simulink model "LAB2_BRUSHED_DC_MOTOR"  (R2023a)
settings: Solver=FixedStepAuto  StartTime=0.0  StopTime=inf  FixedStep=1/200  RelTol=1e-3  EnableMultiTasking=on
undefined symbols (not defined in the file): Dir, ena, freq, LF, pwm
libraries: instrumentseriallib x4, simulink x2, hdlsllib x1
settings Model: PacingRate=10  Creator=User  LastModifiedBy=User
settings SolverCC: AllowMultiTaskInputOutput=on  ConcurrentTasks=on  AutoInsertRateTranBlk=on

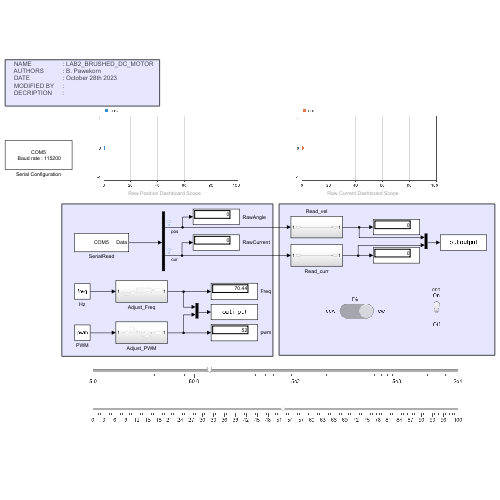
[thumbnail: Simulink's stored preview of the top-level diagram]
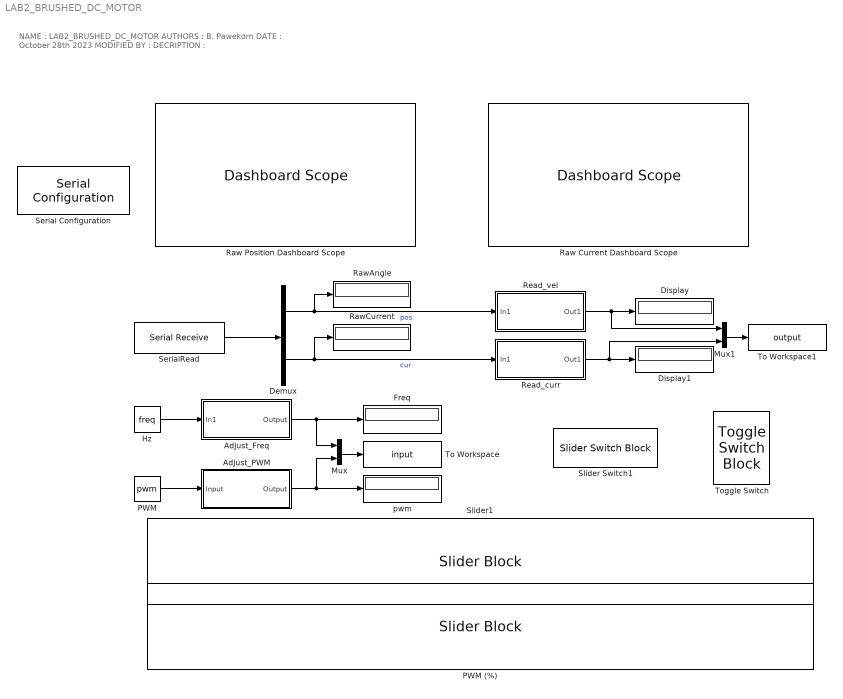
== system LAB2_BRUSHED_DC_MOTOR ==
  note: NAME                  : LAB2_BRUSHED_DC_MOTOR
      |     AUTHORS           : B. Pawekorn
      |     DATE                   : October 28th 2023
      |     MODIFIED BY     :
      |     DECRIPTION      :
  Adjust_Freq : Subsystem
  Adjust_PWM : Subsystem
  Demux : Demux  Outputs=2
  Display : Display
  Display1 : Display
  Freq : Display
  Hz : Constant  Value=freq  OutDataTypeStr=double
  Mux : Mux  Inputs=2
  Mux1 : Mux  Inputs=2
  PWM : Constant  Value=pwm  OutDataTypeStr=uint8
  PWM (%) : SliderBlock  LabelPosition=Hide
  Raw Current Dashboard Scope : DashboardScope  Ymin=0  Ymax=300  UpdateMode=Scroll
  Raw Position Dashboard Scope : DashboardScope  Ymin=0  Ymax=300  UpdateMode=Scroll
  RawAngle : Display
  RawCurrent : Display
  Read_curr : Subsystem
  Read_vel : Subsystem
  Serial Configuration : instrumentseriallib/Serial Configuration  Priority=-200000  PortSel=COM5  Port=COM5  ComPort=COM5  BaudRate=115200  DataBits=8  Parity=none  StopBits=1  ByteOrder=little-endian  FlowControl=none  Timeout=10  SimulateUsing=Interpreted execution  BlockInModel=on  aMode=1
      settings: LibrarySourceBlock=c2000lib/Host Communication/Serial Configuration
  SerialRead : instrumentseriallib/Serial Receive  Priority=1  PortSel=COM5  Port=COM5  ComPort=COM5  DataType=uint16  SaveDataType=uint8  ToggleHeader=on  Header=[69]  ToggleTerminator=on  Terminator=LF ('\n')  CustomTerminator=[]  InputFormat=Column major  ToggleDataSize=on  DataSize=[2]  EnableBlockingMode=on  ActionDataUnavailable=Output last received value  ActionWhenDataUnavailable=Output last received value  CustomValue=0  SampleTime=-1  SimulateUsing=Interpreted execution  BlockInModel=on  aMode=1
  Slider Switch1 : SliderSwitchBlock
      settings: Values={{'ccw', 'cw'}, [1 2]}
  Slider1 : SliderBlock  LabelPosition=Hide  ScaleMin=5  ScaleMax=20000  ScaleType=Log
  To Workspace : ToWorkspace  VariableName=input  SaveFormat=Timeseries  SampleTime=-1
  To Workspace1 : ToWorkspace  VariableName=output  SaveFormat=Timeseries  SampleTime=-1
  Toggle Switch : ToggleSwitchBlock
      settings: Values={{'Off', 'On'}, [0 1]}
  pwm : Display
  wires:
  SerialRead/1 -> Demux/1
  Hz/1 -> Adjust_Freq/1(In1)
  Adjust_PWM/1(Output) -> pwm/1, Mux/2
  Demux/1 -> RawAngle/1, Read_vel/1(In1)  "pos"
  Demux/2 -> RawCurrent/1, Read_curr/1(In1)  "cur"
  PWM/1 -> Adjust_PWM/1(Input)
  Adjust_Freq/1(Output) -> Freq/1, Mux/1
  Read_vel/1(Out1) -> Mux1/1, Display/1
  Read_curr/1(Out1) -> Display1/1, Mux1/2
  Mux/1 -> To Workspace/1
  Mux1/1 -> To Workspace1/1

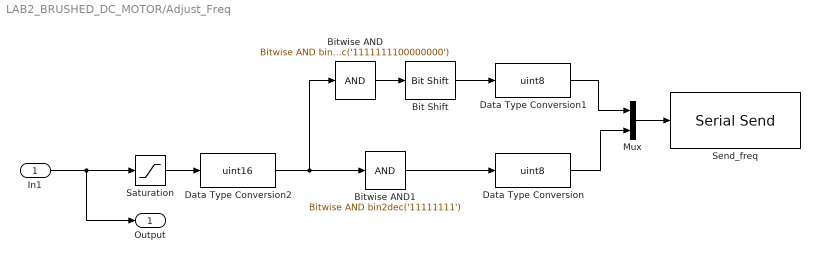
== system LAB2_BRUSHED_DC_MOTOR/Adjust_Freq ==
  In1 : Inport
  Bit Shift : hdlsllib/Logic and Bit Operations/Bit Shift  mode=Shift Right Logical  N=8
  Bitwise AND : simulink/Logic and Bit Operations/Bitwise Operator  logicop=AND  UseBitMask=on  BitMask=bin2dec('1111111100000000')  BitMaskRealWorld=Stored Integer
  Bitwise AND1 : simulink/Logic and Bit Operations/Bitwise Operator  logicop=AND  UseBitMask=on  BitMask=bin2dec('11111111')  BitMaskRealWorld=Stored Integer
  Data Type Conversion : DataTypeConversion  OutDataTypeStr=uint8  SaturateOnIntegerOverflow=off  RndMeth=Floor
  Data Type Conversion1 : DataTypeConversion  OutDataTypeStr=uint8  SaturateOnIntegerOverflow=off  RndMeth=Floor
  Data Type Conversion2 : DataTypeConversion  OutDataTypeStr=uint16  SaturateOnIntegerOverflow=off  RndMeth=Floor
  Mux : Mux  Inputs=2
  Saturation : Saturate  UpperLimit=20000  LowerLimit=5
  Send_freq : instrumentseriallib/Serial Send  Priority=1  PortSel=COM5  Port=COM5  ComPort=COM5  Header=[69]  Terminator=<none>  CustomTerminator=[123]  EnableBlockingMode=on  SimulateUsing=Interpreted execution  BlockInModel=on  aMode=1
  Output : Outport
  wires:
  Mux/1 -> Send_freq/1
  Saturation/1 -> Data Type Conversion2/1
  Data Type Conversion/1 -> Mux/2
  Bitwise AND/1 -> Bit Shift/1
  Bitwise AND1/1 -> Data Type Conversion/1
  Data Type Conversion2/1 -> Bitwise AND1/1, Bitwise AND/1
  Data Type Conversion1/1 -> Mux/1
  Bit Shift/1 -> Data Type Conversion1/1
  In1/1 -> Output/1, Saturation/1

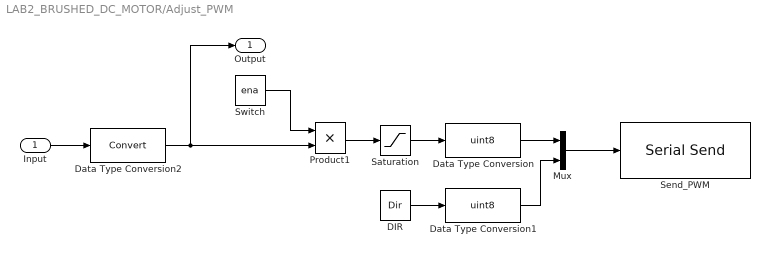
== system LAB2_BRUSHED_DC_MOTOR/Adjust_PWM ==
  Input : Inport
  "DIR " : Constant  Value=Dir
  Data Type Conversion : DataTypeConversion  OutDataTypeStr=uint8  SaturateOnIntegerOverflow=off  RndMeth=Floor
  Data Type Conversion1 : DataTypeConversion  OutDataTypeStr=uint8  SaturateOnIntegerOverflow=off  RndMeth=Floor
  Data Type Conversion2 : DataTypeConversion  SaturateOnIntegerOverflow=off  RndMeth=Floor
  Mux : Mux  Inputs=2
  Product1 : Product
  Saturation : Saturate  UpperLimit=200  LowerLimit=0
  Send_PWM : instrumentseriallib/Serial Send  Priority=1  PortSel=COM5  Port=COM5  ComPort=COM5  Header=[70]  Terminator=<none>  CustomTerminator=[123]  EnableBlockingMode=on  SimulateUsing=Interpreted execution  BlockInModel=on  aMode=1
  Switch : Constant  Value=ena  OutDataTypeStr=uint8
  Output : Outport
  wires:
  Input/1 -> Data Type Conversion2/1
  Switch/1 -> Product1/1
  Product1/1 -> Saturation/1
  Data Type Conversion/1 -> Mux/1
  Saturation/1 -> Data Type Conversion/1
  "DIR "/1 -> Data Type Conversion1/1
  Mux/1 -> Send_PWM/1
  Data Type Conversion1/1 -> Mux/2
  Data Type Conversion2/1 -> Output/1, Product1/2

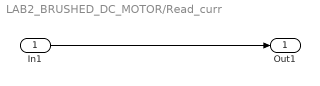
== system LAB2_BRUSHED_DC_MOTOR/Read_curr ==
  In1 : Inport
  Out1 : Outport
  wires:
  In1/1 -> Out1/1

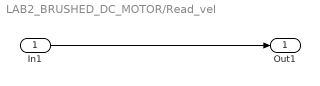
== system LAB2_BRUSHED_DC_MOTOR/Read_vel ==
  In1 : Inport
  Out1 : Outport
  wires:
  In1/1 -> Out1/1
